simulink model "wash_out_filter_previous_version"  (R2021b)
settings: Solver=FixedStepAuto  StartTime=0.0  StopTime=100  FixedStep=0.01  RelTol=1e-3
values from neighbouring files (symbols this model uses):
  Kroll = rollGrad*pi/180    (= 0.0715584993318)    [Init_for_washout_filter.m]
  rx = 0.29    [Init_for_washout_filter.m]    (also in UKF_start.m)
  T = 0.15    [Init_for_washout_filter.m]
  threshold_vx = 1    [Init_for_washout_filter.m]
  Ts = 0.01    [Init_for_washout_filter.m]    (also in UKF_start.m)
settings Model: Creator=thomasperrein  LastModifiedBy=thomasperrein
settings SolverCC: AlgebraicLoopSolver=TrustRegion
settings DebuggingCC: ArithmeticOperatorsInVariantConditions=warning
settings SFSimCC: CustomCodeUndefinedFunction=UseInterfaceOnly

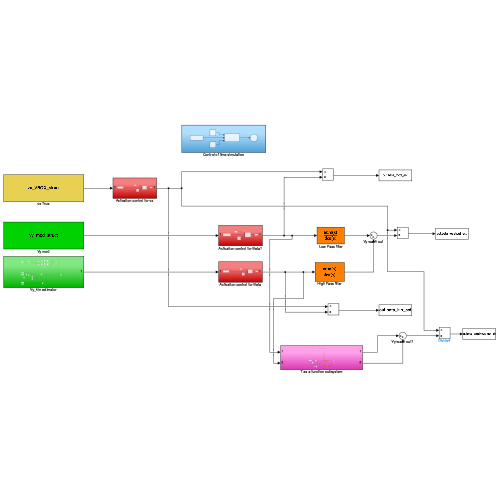
[thumbnail: Simulink's stored preview of the top-level diagram]
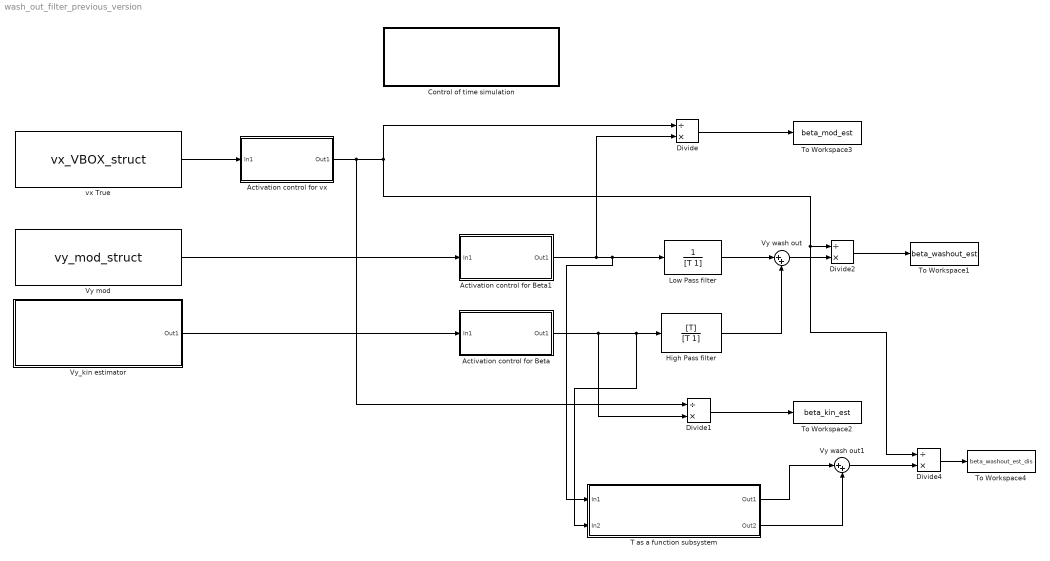
== system wash_out_filter_previous_version ==
  " Low Pass filter" : TransferFcn  Denominator=[T 1]
  Activation control for Beta : Subsystem
  Activation control for Beta1 : Subsystem
  Activation control for vx : Subsystem
  Control of time simulation : Subsystem
  Divide{,1..2,4} (4 alike) : Product  Inputs=/*
  High Pass filter : TransferFcn  Numerator=[T]  Denominator=[T 1]
  T as a function subsystem : Subsystem
  To Workspace1 : ToWorkspace  VariableName=beta_washout_est  SaveFormat=Timeseries  SampleTime=-1
  To Workspace2 : ToWorkspace  VariableName=beta_kin_est  SaveFormat=Timeseries  SampleTime=-1
  To Workspace3 : ToWorkspace  VariableName=beta_mod_est  SaveFormat=Timeseries  SampleTime=-1
  To Workspace4 : ToWorkspace  VariableName=beta_washout_est_dis  SaveFormat=Timeseries  SampleTime=-1
  Vy mod : FromWorkspace  VariableName=vy_mod_struct
  Vy wash out : Sum  Inputs=|++
  Vy wash out1 : Sum  Inputs=|++
  Vy_kin estimator : Subsystem
  vx True : FromWorkspace  VariableName=vx_VBOX_struct
  wires:
  Vy mod/1 -> Activation control for Beta1/1(In1)
  " Low Pass filter"/1 -> Vy wash out/1
  High Pass filter/1 -> Vy wash out/2
  Vy_kin estimator/1(Out1) -> Activation control for Beta/1(In1)
  Activation control for Beta/1(Out1) -> Divide1/2, T as a function subsystem/2(In2), High Pass filter/1
  Vy wash out/1 -> Divide2/2
  Activation control for Beta1/1(Out1) -> Divide/2, T as a function subsystem/1(In1), " Low Pass filter"/1
  vx True/1 -> Activation control for vx/1(In1)
  Divide1/1 -> To Workspace2/1
  Divide/1 -> To Workspace3/1
  Divide2/1 -> To Workspace1/1
  Activation control for vx/1(Out1) -> Divide1/1, Divide4/1, Divide2/1, Divide/1
  Vy wash out1/1 -> Divide4/2
  Divide4/1 -> To Workspace4/1
  T as a function subsystem/1(Out1) -> Vy wash out1/1
  T as a function subsystem/2(Out2) -> Vy wash out1/2

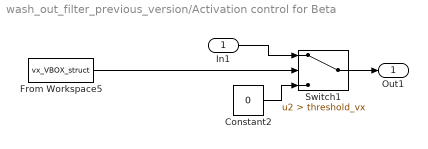
== system wash_out_filter_previous_version/Activation control for Beta ==
  In1 : Inport
  Constant2 : Constant  Value=0
  From Workspace5 : FromWorkspace  VariableName=vx_VBOX_struct
  Switch1 : Switch  Criteria=u2 > Threshold  Threshold=threshold_vx
  Out1 : Outport
  wires:
  Switch1/1 -> Out1/1
  In1/1 -> Switch1/1
  Constant2/1 -> Switch1/3
  From Workspace5/1 -> Switch1/2

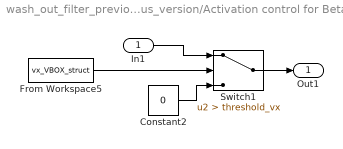
== system wash_out_filter_previous_version/Activation control for Beta1 ==
  In1 : Inport
  Constant2 : Constant  Value=0
  From Workspace5 : FromWorkspace  VariableName=vx_VBOX_struct
  Switch1 : Switch  Criteria=u2 > Threshold  Threshold=threshold_vx
  Out1 : Outport
  wires:
  Switch1/1 -> Out1/1
  In1/1 -> Switch1/1
  Constant2/1 -> Switch1/3
  From Workspace5/1 -> Switch1/2

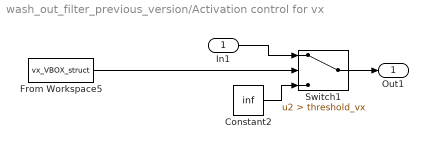
== system wash_out_filter_previous_version/Activation control for vx ==
  In1 : Inport
  Constant2 : Constant  Value=inf
  From Workspace5 : FromWorkspace  VariableName=vx_VBOX_struct
  Switch1 : Switch  Criteria=u2 > Threshold  Threshold=threshold_vx
  Out1 : Outport
  wires:
  Switch1/1 -> Out1/1
  In1/1 -> Switch1/1
  Constant2/1 -> Switch1/3
  From Workspace5/1 -> Switch1/2

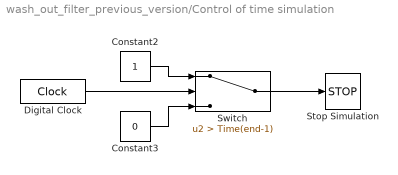
== system wash_out_filter_previous_version/Control of time simulation ==
  Constant2 : Constant
  Constant3 : Constant  Value=0
  Digital Clock : DigitalClock  SampleTime=0.01
  Stop Simulation : Stop
  Switch : Switch  Criteria=u2 > Threshold  Threshold=Time(end-1)
  wires:
  Constant3/1 -> Switch/3
  Constant2/1 -> Switch/1
  Switch/1 -> Stop Simulation/1
  Digital Clock/1 -> Switch/2

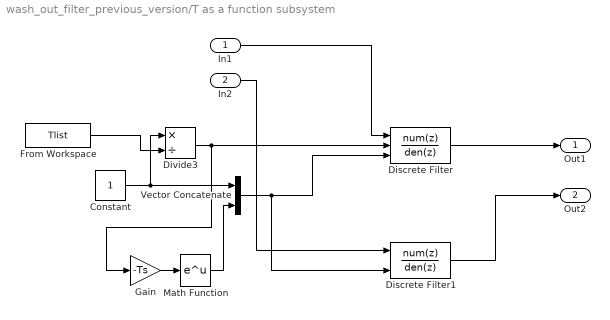
== system wash_out_filter_previous_version/T as a function subsystem ==
  In1 : Inport
  In2 : Inport  Port=2
  Constant : Constant
  Discrete Filter : DiscreteFilter  NumeratorSource=Input port  DenominatorSource=Input port  a0EqualsOne=on
      settings: InputPortMap=u0,p1,p3
  Discrete Filter1 : DiscreteFilter  DenominatorSource=Input port  a0EqualsOne=on
      settings: InputPortMap=u0,p3
  Divide3 : Product  Inputs=*/
  From Workspace : FromWorkspace  VariableName=Tlist
  Gain : Gain  Gain=-Ts
  Math Function : Math  SaturateOnIntegerOverflow=on
  Vector Concatenate : Concatenate
  Out1 : Outport
  Out2 : Outport  Port=2
  wires:
  Discrete Filter1/1 -> Out2/1
  Gain/1 -> Math Function/1
  Vector Concatenate/1 -> Discrete Filter1/2, Discrete Filter/3
  In2/1 -> Discrete Filter1/1
  Math Function/1 -> Vector Concatenate/2
  In1/1 -> Discrete Filter/1
  Divide3/1 -> Gain/1, Discrete Filter/2
  From Workspace/1 -> Divide3/2
  Discrete Filter/1 -> Out1/1
  Constant/1 -> Vector Concatenate/1, Divide3/1

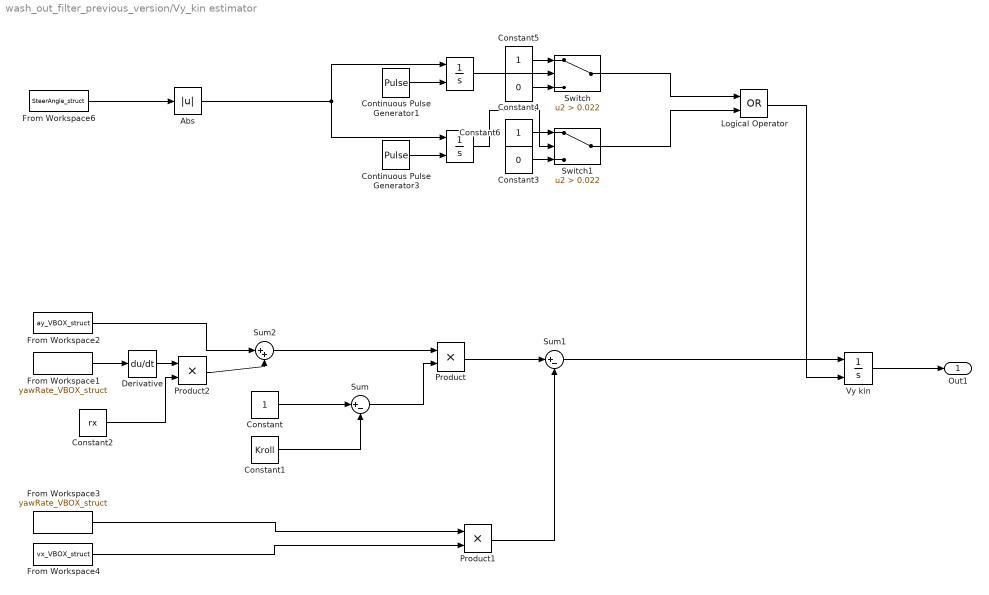
== system wash_out_filter_previous_version/Vy_kin estimator ==
  " " : Integrator  ExternalReset=rising
  " " : Integrator  ExternalReset=rising
  Abs : Abs
  Constant : Constant
  Constant1 : Constant  Value=Kroll
  Constant2 : Constant  Value=rx
  Constant3 : Constant  Value=0
  Constant4 : Constant  Value=0
  Constant5 : Constant
  Constant6 : Constant
  Continuous Pulse Generator1 : DiscretePulseGenerator  PulseType=Time based  Period=4  PulseWidth=50
  Continuous Pulse Generator3 : DiscretePulseGenerator  PulseType=Time based  Period=4  PulseWidth=50  PhaseDelay=4/2
  Derivative : Derivative
  From Workspace1 : FromWorkspace  VariableName=yawRate_VBOX_struct
  From Workspace2 : FromWorkspace  VariableName=ay_VBOX_struct
  From Workspace3 : FromWorkspace  VariableName=yawRate_VBOX_struct
  From Workspace4 : FromWorkspace  VariableName=vx_VBOX_struct
  From Workspace6 : FromWorkspace  VariableName=SteerAngle_struct
  Logical Operator : Logic  Operator=OR  AllPortsSameDT=off  OutDataTypeStr=boolean
  Product : Product
  Product1 : Product
  Product2 : Product
  Sum : Sum  Inputs=|+-
  Sum1 : Sum  Inputs=|+-
  Sum2 : Sum  Inputs=|++
  Switch : Switch  Criteria=u2 > Threshold  Threshold=0.022
  Switch1 : Switch  Criteria=u2 > Threshold  Threshold=0.022
  Vy kin : Integrator  ExternalReset=rising
  Out1 : Outport
  wires:
  From Workspace3/1 -> Product1/1
  Constant1/1 -> Sum/2
  Product/1 -> Sum1/1
  Sum/1 -> Product/2
  Constant/1 -> Sum/1
  Product1/1 -> Sum1/2
  Vy kin/1 -> Out1/1
  From Workspace4/1 -> Product1/2
  From Workspace1/1 -> Derivative/1
  Derivative/1 -> Product2/1
  Constant2/1 -> Product2/2
  Product2/1 -> Sum2/2
  Sum2/1 -> Product/1
  From Workspace2/1 -> Sum2/1
  Sum1/1 -> Vy kin/1
  Constant5/1 -> Switch/1
  Constant4/1 -> Switch/3
  From Workspace6/1 -> Abs/1
  Constant3/1 -> Switch1/3
  Constant6/1 -> Switch1/1
  Abs/1 -> " "/1, " "/1
  Switch1/1 -> Logical Operator/2
  Switch/1 -> Logical Operator/1
  " "/1 -> Switch/2
  " "/1 -> Switch1/2
  Continuous Pulse Generator1/1 -> " "/2
  Continuous Pulse Generator3/1 -> " "/2
  Logical Operator/1 -> Vy kin/2
